simulink model "Simulationsprojekt_PWM_Vorlage"  (R2024b)
settings: Solver=ode45  StartTime=0.0  StopTime=0.005  FixedStep=0.5*T_PWM  MaxStep=2e-6  RelTol=1e-3
InitFcn:
  | run Init_Simulationsprojekt_PWM.m
values from neighbouring files (symbols this model uses):
  f_elec = 500    [Init_Simulationsprojekt_PWM.m]
  m_max = 2/sqrt(3)    [Init_Simulationsprojekt_PWM.m]
  T_PWM = 1/f_switching    (= 0.0001)    [Init_Simulationsprojekt_PWM.m]
  u_d = -0.8*(U_DC/2*m_max)    [Init_Simulationsprojekt_PWM.m]
  U_DC = 800    [Init_Simulationsprojekt_PWM.m]
  u_q = 0.5*(U_DC/2*m_max)    [Init_Simulationsprojekt_PWM.m]
libraries: simulink x3
settings Model: Creator=PAKUNER  LastModifiedBy=Jan Tepel
settings SolverCC: AlgebraicLoopSolver=TrustRegion
settings DebuggingCC: UnconnectedInputMsg=warning  UnconnectedOutputMsg=warning  UnconnectedLineMsg=warning
settings ModelReferenceCC: EnableRefExpFcnMdlSchedulingChecks=on
settings RTWCC: GPUComputeCapability=3.5  DLArmComputeVersion=19.05

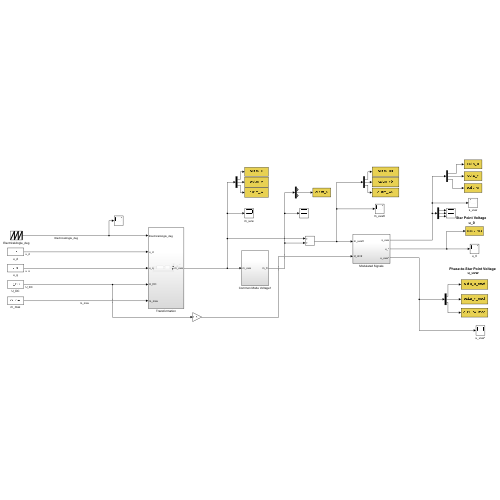
[thumbnail: Simulink's stored preview of the top-level diagram]
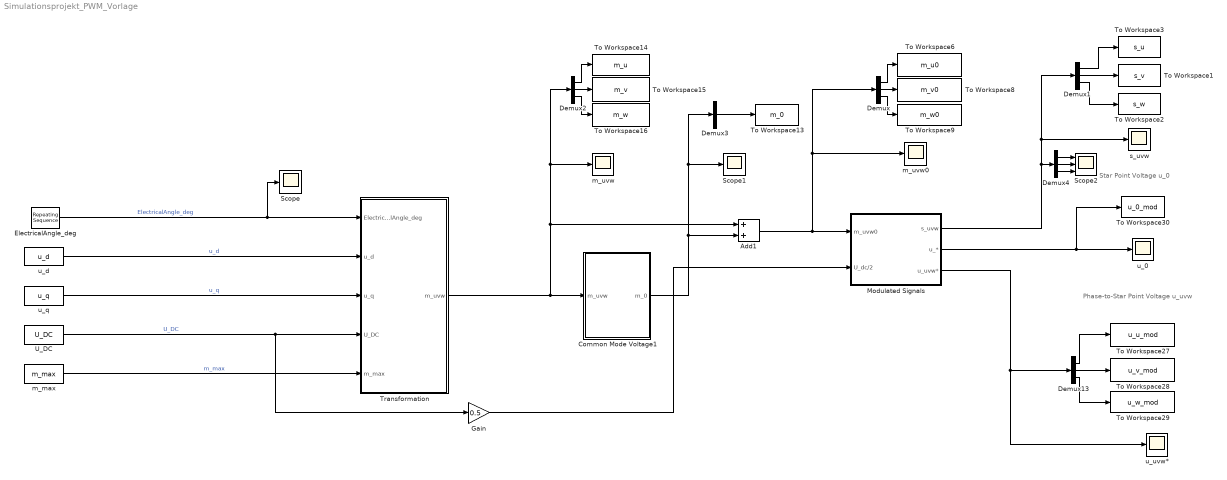
== system Simulationsprojekt_PWM_Vorlage ==
  note: Phase-to-Star Point Voltage
      | u_uvw
  note: Star Point Voltage
      | u_0
  Add1 : Sum
  Common Mode Voltage1 : Subsystem
  Demux{,1..4,13} (6 alike) : Demux  Outputs=3
  ElectricalAngle_deg : simulink/Sources/Repeating Sequence  rep_seq_t=[0 1/f_elec]  rep_seq_y=[0 360]
  Gain : Gain  Gain=0.5
  Modulated Signals : Subsystem  StartFcn=run Init_Simulationsprojekt_PWM.m
  Scope : Scope
  Scope1 : Scope
  Scope2 : Scope  NumInputPorts=3
  To Workspace1 : ToWorkspace  VariableName=s_v  SampleTime=-1
  To Workspace13 : ToWorkspace  VariableName=m_0  SampleTime=-1
  To Workspace14 : ToWorkspace  VariableName=m_u  SampleTime=-1
  To Workspace15 : ToWorkspace  VariableName=m_v  SampleTime=-1
  To Workspace16 : ToWorkspace  VariableName=m_w  SampleTime=-1
  To Workspace2 : ToWorkspace  VariableName=s_w  SampleTime=-1
  To Workspace27 : ToWorkspace  VariableName=u_u_mod  SampleTime=-1
  To Workspace28 : ToWorkspace  VariableName=u_v_mod  SampleTime=-1
  To Workspace29 : ToWorkspace  VariableName=u_w_mod  SampleTime=-1
  To Workspace3 : ToWorkspace  VariableName=s_u  SampleTime=-1
  To Workspace30 : ToWorkspace  VariableName=u_0_mod  SampleTime=-1
  To Workspace6 : ToWorkspace  VariableName=m_u0  SampleTime=-1
  To Workspace8 : ToWorkspace  VariableName=m_v0  SampleTime=-1
  To Workspace9 : ToWorkspace  VariableName=m_w0  SampleTime=-1
  Transformation : Subsystem
  U_DC : Constant  Value=U_DC
  m_max : Constant  Value=m_max
  m_uvw : Scope
  m_uvw0 : Scope
  s_uvw : Scope
  u_0 : Scope
  u_d : Constant  Value=u_d
  u_q : Constant  Value=u_q
  u_uvw* : Scope
  wires:
  Demux2/3 -> To Workspace16/1
  Demux2/1 -> To Workspace14/1
  Demux2/2 -> To Workspace15/1
  Demux/1 -> To Workspace6/1
  Demux/2 -> To Workspace8/1
  Demux/3 -> To Workspace9/1
  Add1/1 -> Demux/1, m_uvw0/1, Modulated Signals/1(m_uvw0)
  Transformation/1(m_uvw) -> m_uvw/1, Demux2/1, Add1/1, Common Mode Voltage1/1(m_uvw)
  ElectricalAngle_deg/1 -> Scope/1, Transformation/1(ElectricalAngle_deg)  "ElectricalAngle_deg"
  u_d/1 -> Transformation/2(u_d)  "u_d"
  u_q/1 -> Transformation/3(u_q)  "u_q"
  U_DC/1 -> Gain/1, Transformation/4(U_DC)  "U_DC"
  m_max/1 -> Transformation/5(m_max)  "m_max"
  Gain/1 -> Modulated Signals/2(U_dc/2)
  Common Mode Voltage1/1(m_0) -> Scope1/1, Demux3/1, Add1/2
  Demux1/3 -> To Workspace2/1
  Demux1/1 -> To Workspace3/1
  Modulated Signals/1(s_uvw) -> Demux4/1, Demux1/1, s_uvw/1
  Demux1/2 -> To Workspace1/1
  Demux13/3 -> To Workspace29/1
  Demux13/1 -> To Workspace27/1
  Demux13/2 -> To Workspace28/1
  Modulated Signals/3(u_uvw*) -> Demux13/1, u_uvw*/1
  Modulated Signals/2(u_*) -> To Workspace30/1, u_0/1
  Demux3/2 -> To Workspace13/1
  Demux4/1 -> Scope2/1
  Demux4/2 -> Scope2/2
  Demux4/3 -> Scope2/3

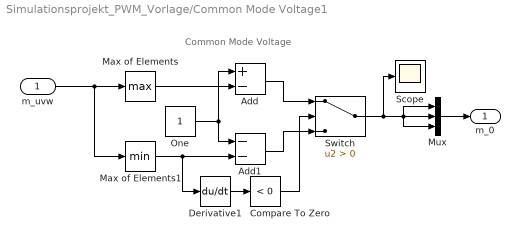
== system Simulationsprojekt_PWM_Vorlage/Common Mode Voltage1 ==
  note: Common Mode Voltage
  m_uvw : Inport
  Add : Sum  Inputs=+-
  Add1 : Sum  Inputs=--
  Compare To Zero : simulink/Logic and Bit Operations/Compare To Zero  relop=<  OutDataTypeStr=boolean
  Derivative1 : Derivative
  Max of Elements : MinMax  Function=max
  Max of Elements1 : MinMax
  Mux : Mux  Inputs=3
  One : Constant  OutDataTypeStr=Inherit: Inherit via back propagation
  Scope : Scope
  Switch : Switch  Criteria=u2 > Threshold  SaturateOnIntegerOverflow=off  InputSameDT=off
  m_0 : Outport
  wires:
  Switch/1 -> Mux/1, Mux/3, Mux/2, Scope/1
  Max of Elements1/1 -> Add1/2, Derivative1/1
  One/1 -> Add/1, Add1/1
  Mux/1 -> m_0/1
  Add/1 -> Switch/1
  Add1/1 -> Switch/3
  Derivative1/1 -> Compare To Zero/1
  Compare To Zero/1 -> Switch/2
  m_uvw/1 -> Max of Elements1/1, Max of Elements/1
  Max of Elements/1 -> Add/2

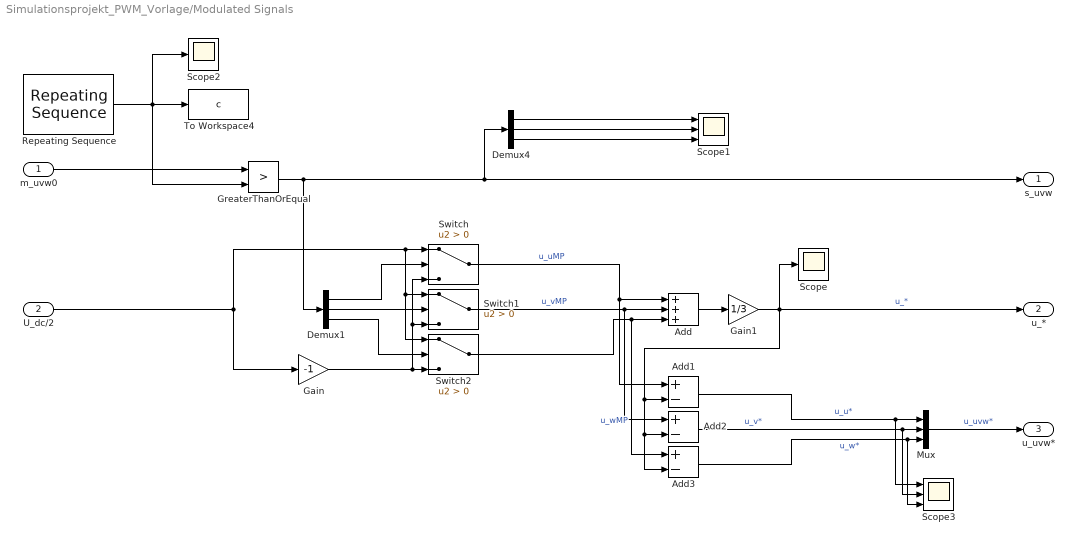
== system Simulationsprojekt_PWM_Vorlage/Modulated Signals ==
  m_uvw0 : Inport
  U_dc/2 : Inport  Port=2
  Add : Sum  Inputs=+++
  Add1 : Sum  Inputs=+-
  Add2 : Sum  Inputs=+-
  Add3 : Sum  Inputs=+-
  Demux1 : Demux  Outputs=3
  Demux4 : Demux  Outputs=3
  Gain : Gain  Gain=-1
  Gain1 : Gain  Gain=1/3
  GreaterThanOrEqual : RelationalOperator  Operator=>  OutDataTypeStr=boolean  RndMeth=Simplest  InputSameDT=off
  Mux : Mux  Inputs=3
  Repeating Sequence : simulink/Sources/Repeating Sequence  rep_seq_t=[0 T_PWM/2 T_PWM]  rep_seq_y=[-1 1 -1]
  Scope : Scope
  Scope1 : Scope  NumInputPorts=3
  Scope2 : Scope
  Scope3 : Scope  NumInputPorts=3
  Switch : Switch  Criteria=u2 > Threshold  SaturateOnIntegerOverflow=off  InputSameDT=off
  Switch1 : Switch  Criteria=u2 > Threshold  SaturateOnIntegerOverflow=off  InputSameDT=off
  Switch2 : Switch  Criteria=u2 > Threshold  SaturateOnIntegerOverflow=off  InputSameDT=off
  To Workspace4 : ToWorkspace  VariableName=c  SampleTime=-1
  s_uvw : Outport
  u_* : Outport  Port=2
  u_uvw* : Outport  Port=3
  wires:
  Repeating Sequence/1 -> GreaterThanOrEqual/2, Scope2/1, To Workspace4/1
  m_uvw0/1 -> GreaterThanOrEqual/1
  Demux4/2 -> Scope1/2
  Demux4/1 -> Scope1/1
  Demux4/3 -> Scope1/3
  GreaterThanOrEqual/1 -> Demux1/1, Demux4/1, s_uvw/1
  Demux1/1 -> Switch/2
  Demux1/2 -> Switch1/2
  Demux1/3 -> Switch2/2
  Gain/1 -> Switch/3, Switch1/3, Switch2/3
  Switch1/1 -> Add2/1, Add/2  "u_vMP"
  Switch2/1 -> Add3/1, Add/3  "u_wMP"
  Add/1 -> Gain1/1
  Gain1/1 -> u_*/1, Add1/2, Add2/2, Add3/2, Scope/1  "u_*"
  Switch/1 -> Add1/1, Add/1  "u_uMP"
  Add1/1 -> Scope3/1, Mux/1  "u_u*"
  Add2/1 -> Scope3/2, Mux/2  "u_v*"
  Add3/1 -> Scope3/3, Mux/3  "u_w*"
  Mux/1 -> u_uvw*/1  "u_uvw*"
  U_dc/2/1 -> Gain/1, Switch1/1, Switch2/1, Switch/1

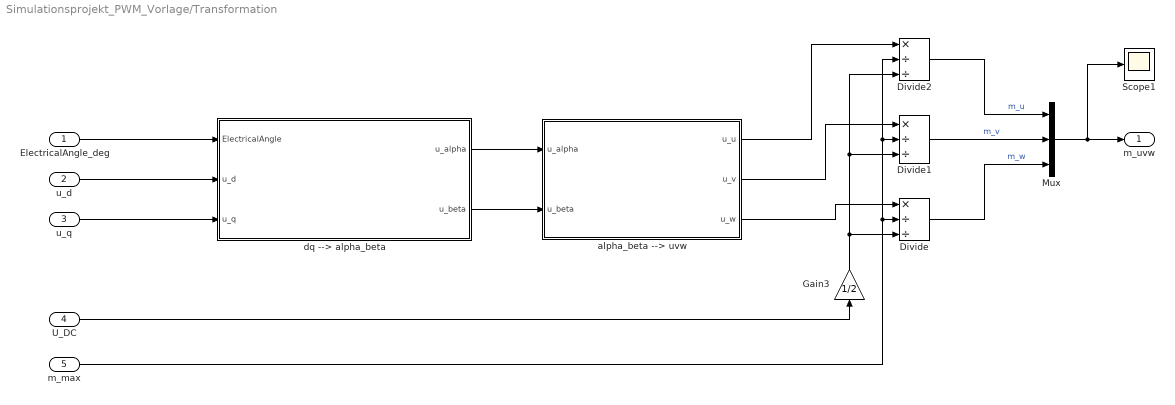
== system Simulationsprojekt_PWM_Vorlage/Transformation ==
  ElectricalAngle_deg : Inport
  u_d : Inport  Port=2
  u_q : Inport  Port=3
  U_DC : Inport  Port=4
  m_max : Inport  Port=5
  Divide : Product  Inputs=*//
  Divide1 : Product  Inputs=*//
  Divide2 : Product  Inputs=*//
  Gain3 : Gain  Gain=1/2
  Mux : Mux  Inputs=3
  Scope1 : Scope
  alpha_beta --> uvw : Subsystem
  dq --> alpha_beta : Subsystem
  m_uvw : Outport
  wires:
  Mux/1 -> Scope1/1, m_uvw/1
  U_DC/1 -> Gain3/1
  Gain3/1 -> Divide1/3, Divide2/3, Divide/3
  Divide1/1 -> Mux/2  "m_v"
  Divide/1 -> Mux/3  "m_w"
  Divide2/1 -> Mux/1  "m_u"
  m_max/1 -> Divide2/2, Divide1/2, Divide/2
  ElectricalAngle_deg/1 -> dq --> alpha_beta/1(ElectricalAngle)
  u_d/1 -> dq --> alpha_beta/2(u_d)
  u_q/1 -> dq --> alpha_beta/3(u_q)
  dq --> alpha_beta/1(u_alpha) -> alpha_beta --> uvw/1(u_alpha)
  dq --> alpha_beta/2(u_beta) -> alpha_beta --> uvw/2(u_beta)
  alpha_beta --> uvw/1(u_u) -> Divide2/1
  alpha_beta --> uvw/2(u_v) -> Divide1/1
  alpha_beta --> uvw/3(u_w) -> Divide/1

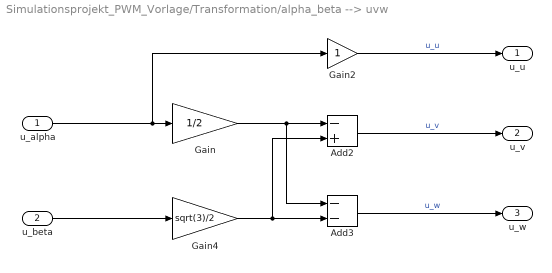
== system Simulationsprojekt_PWM_Vorlage/Transformation/alpha_beta --> uvw ==
  u_alpha : Inport
  u_beta : Inport  Port=2
  Add2 : Sum  Inputs=-+
  Add3 : Sum  Inputs=--
  Gain : Gain  Gain=1/2
  Gain2 : Gain
  Gain4 : Gain  Gain=sqrt(3)/2
  u_u : Outport
  u_v : Outport  Port=2
  u_w : Outport  Port=3
  wires:
  Gain/1 -> Add3/1, Add2/1
  u_beta/1 -> Gain4/1
  Gain2/1 -> u_u/1  "u_u"
  Gain4/1 -> Add3/2, Add2/2
  u_alpha/1 -> Gain2/1, Gain/1
  Add2/1 -> u_v/1  "u_v"
  Add3/1 -> u_w/1  "u_w"

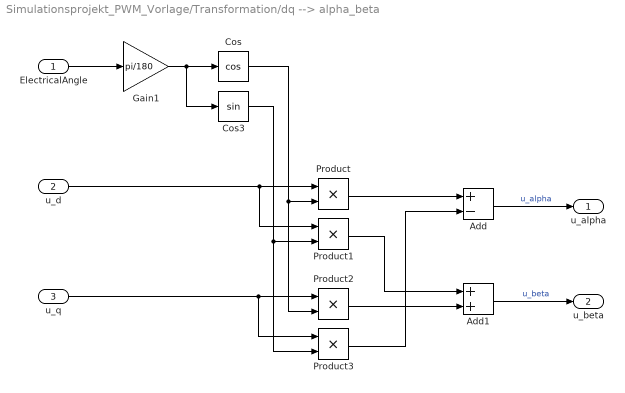
== system Simulationsprojekt_PWM_Vorlage/Transformation/dq --> alpha_beta ==
  ElectricalAngle : Inport
  u_d : Inport  Port=2
  u_q : Inport  Port=3
  Add : Sum  Inputs=+-
  Add1 : Sum
  Cos : Trigonometry  Operator=cos
  Cos3 : Trigonometry
  Gain1 : Gain  Gain=pi/180
  Product{,1..3} (4 alike) : Product
  u_alpha : Outport
  u_beta : Outport  Port=2
  wires:
  u_q/1 -> Product3/1, Product2/1
  Add1/1 -> u_beta/1  "u_beta"
  Product1/1 -> Add1/1
  Product3/1 -> Add/2
  Add/1 -> u_alpha/1  "u_alpha"
  Cos3/1 -> Product3/2, Product1/2
  Cos/1 -> Product2/2, Product/2
  Product2/1 -> Add1/2
  Gain1/1 -> Cos3/1, Cos/1
  Product/1 -> Add/1
  u_d/1 -> Product/1, Product1/1
  ElectricalAngle/1 -> Gain1/1
